simulink model "internalights"  (R2020b)
settings: Solver=FixedStepAuto  StartTime=0.0  StopTime=10  FixedStep=0.1  RelTol=1e-3
undefined symbols (not defined in the file): sigbuilder_block
libraries: simulink x4
settings Model: NumberOfSteps=10  Creator=training  LastModifiedBy=training

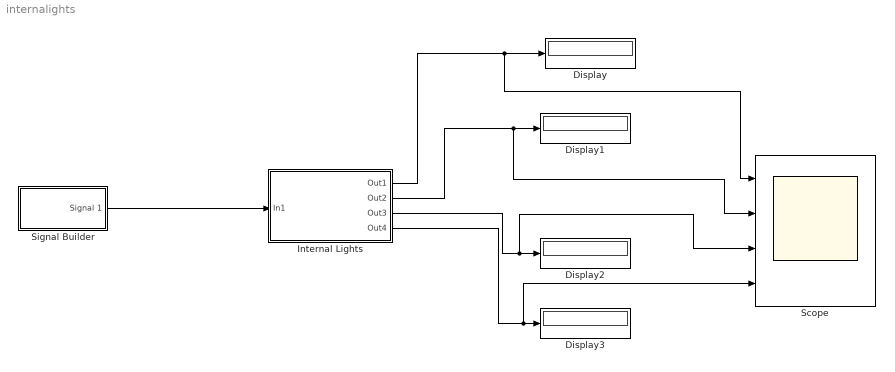
== system internalights ==
  Display{,1..3} (4 alike) : Display
  Internal Lights : Subsystem
  Scope : Scope  NumInputPorts=4
  Signal Builder : Subsystem  Tag=STV Subsys  LoadFcn=sigbuilder_block('load');  StartFcn=sigbuilder_block('start');  StopFcn=sigbuilder_block('stop');  ClipboardFcn=sigbuilder_block('clipboard');  mask(Sigbuilder block){tuvar=[0:10]}
      mask help: Simulink:masks:SigbuilderBlock_MD
      mask init:
      | if ~strcmp(get_param(bdroot(gcbh),'SimulationStatus'),'stopped') tuvar = sigbuilder_block('maskInit'); end
      settings: CopyFcn=sigbuilder_block('copy');  DeleteFcn=sigbuilder_block('delete');  ModelCloseFcn=sigbuilder_block('modelClose');  PreSaveFcn=sigbuilder_block('preSave');  PauseFcn=sigbuilder_block('pause');  ContinueFcn=sigbuilder_block('continue');  NameChangeFcn=sigbuilder_block('namechange');  OpenFcn=sigbuilder_block('open',[437.6 153 550.4 359.25 ]);  CloseFcn=sigbuilder_block('close');
      mask Display: plot(0, 0, 100, 100,[2, 2, 32, 32, 2], [68, 8, 8, 68, 68],[32, 2], [38, 38], [32, 19, 2],[53, 60, 44], [32, 17, 17, 2],[16, 16, 31, 31]);txt = getActiveGroup(gcbh);text(2, 100, txt,'verticalAlignment', 'top');
  wires:
  Signal Builder/1(Signal 1) -> Internal Lights/1(In1)
  Internal Lights/1(Out1) -> Scope/1, Display/1
  Internal Lights/2(Out2) -> Scope/2, Display1/1
  Internal Lights/3(Out3) -> Scope/3, Display2/1
  Internal Lights/4(Out4) -> Scope/4, Display3/1

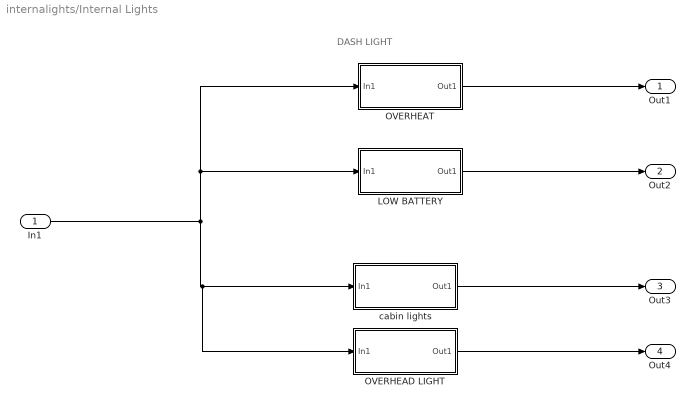
== system internalights/Internal Lights ==
  note: DASH LIGHT
  In1 : Inport
  LOW BATTERY : Subsystem
  OVERHEAD LIGHT : Subsystem
  OVERHEAT : Subsystem
  cabin lights : Subsystem
  Out1 : Outport
  Out2 : Outport  Port=2
  Out3 : Outport  Port=3
  Out4 : Outport  Port=4
  wires:
  In1/1 -> OVERHEAD LIGHT/1(In1), cabin lights/1(In1), LOW BATTERY/1(In1), OVERHEAT/1(In1)
  OVERHEAT/1(Out1) -> Out1/1
  LOW BATTERY/1(Out1) -> Out2/1
  OVERHEAD LIGHT/1(Out1) -> Out4/1
  cabin lights/1(Out1) -> Out3/1

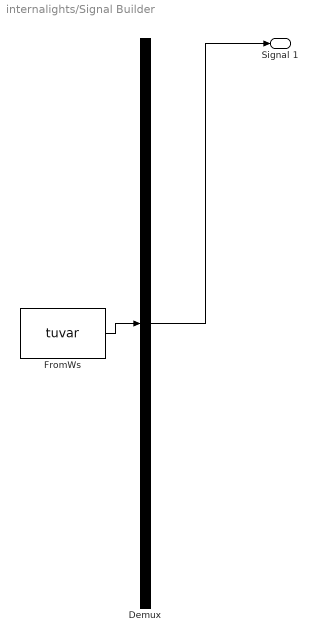
== system internalights/Signal Builder ==
  Demux : Demux  Tag=STV Demux  Outputs=1
      settings: DisplayOption=none
  FromWs : FromWorkspace  Tag=STV FromWs  VariableName=tuvar
      SigBuilderData=|
      | common.afterFinalStr = 'Extrapolate'
      | common.sampleTime = 0
      | dataSet.timeRange = [0 10]
      | dataSet.name = 'Group 1'
      | sbobj.Groups.Name = 'Group 1'
      | sbobj.Groups.Signals.Name = 'Signal 1'
      | sbobj.Groups.Signals.XData = [0 4 4 6 6 10]
      | sbobj.Groups.Signals.YData = [0 0 1 1 0 0]
  Signal 1 : Outport  Tag=STV Outport
  wires:
  Demux/1 -> Signal 1/1
  FromWs/1 -> Demux/1

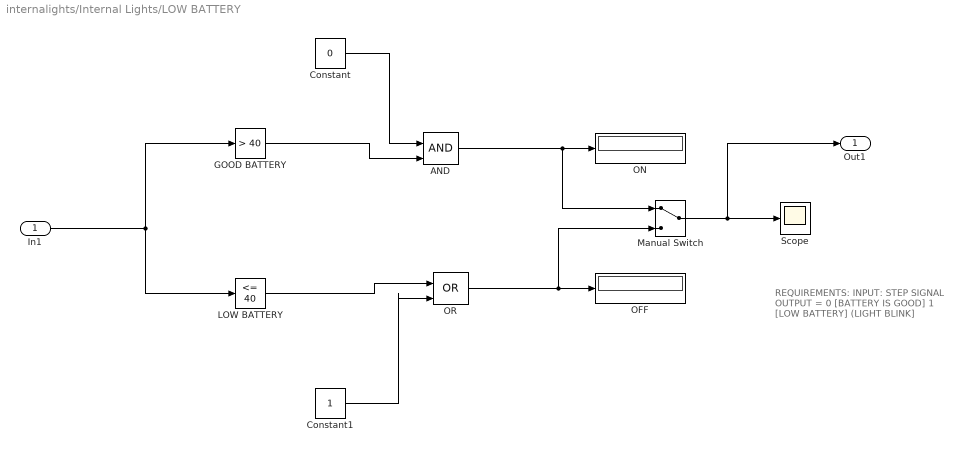
== system internalights/Internal Lights/LOW BATTERY ==
  note: REQUIREMENTS:
      | INPUT: STEP SIGNAL
      | OUTPUT = 0 [BATTERY IS GOOD]
      | 1 [LOW BATTERY] (LIGHT BLINK]
  In1 : Inport
  AND : Logic  IconShape=distinctive  AllPortsSameDT=off  OutDataTypeStr=boolean
  Constant : Constant  Value=0
  Constant1 : Constant
  GOOD BATTERY : simulink/Logic and Bit Operations/Compare To Constant  relop=>  const=40  OutDataTypeStr=boolean
  LOW BATTERY : simulink/Logic and Bit Operations/Compare To Constant  relop=<=  const=40  OutDataTypeStr=boolean
  Manual Switch : ManualSwitch
  OFF : Display
  ON : Display
  OR : Logic  Operator=OR  IconShape=distinctive  AllPortsSameDT=off  OutDataTypeStr=boolean
  Scope : Scope
  Out1 : Outport
  wires:
  OR/1 -> Manual Switch/2, OFF/1
  AND/1 -> Manual Switch/1, ON/1
  Manual Switch/1 -> Out1/1, Scope/1
  Constant1/1 -> OR/2
  GOOD BATTERY/1 -> AND/2
  Constant/1 -> AND/1
  LOW BATTERY/1 -> OR/1
  In1/1 -> LOW BATTERY/1, GOOD BATTERY/1

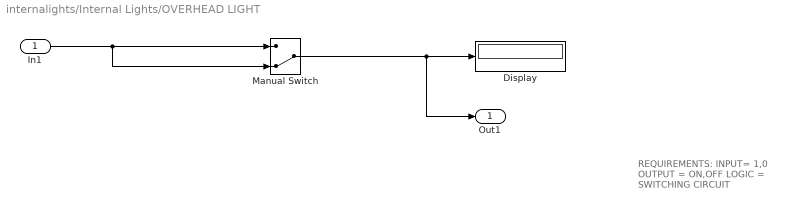
== system internalights/Internal Lights/OVERHEAD LIGHT ==
  note: REQUIREMENTS:
      | INPUT= 1,0
      | OUTPUT = ON,OFF
      | LOGIC = SWITCHING CIRCUIT
  In1 : Inport
  Display : Display
  Manual Switch : ManualSwitch  CurrentSetting=0
  Out1 : Outport
  wires:
  In1/1 -> Manual Switch/2, Manual Switch/1
  Manual Switch/1 -> Out1/1, Display/1

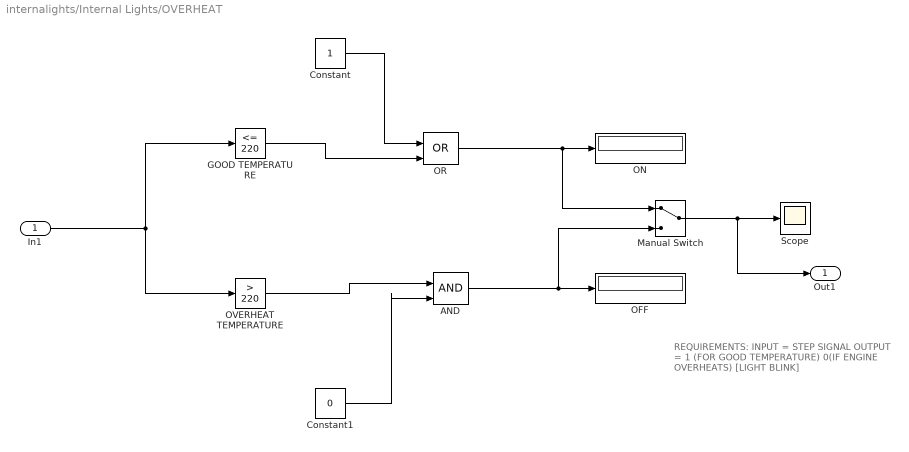
== system internalights/Internal Lights/OVERHEAT ==
  note: REQUIREMENTS:
      | INPUT = STEP SIGNAL
      | OUTPUT = 1 (FOR GOOD TEMPERATURE)
      | 0(IF ENGINE OVERHEATS) [LIGHT BLINK]
  In1 : Inport
  AND : Logic  IconShape=distinctive  AllPortsSameDT=off  OutDataTypeStr=boolean
  Constant : Constant
  Constant1 : Constant  Value=0
  GOOD TEMPERATURE : simulink/Logic and Bit Operations/Compare To Constant  relop=<=  const=220  OutDataTypeStr=boolean
  Manual Switch : ManualSwitch
  OFF : Display
  ON : Display
  OR : Logic  Operator=OR  IconShape=distinctive  AllPortsSameDT=off  OutDataTypeStr=boolean
  OVERHEAT TEMPERATURE : simulink/Logic and Bit Operations/Compare To Constant  relop=>  const=220  OutDataTypeStr=boolean
  Scope : Scope
  Out1 : Outport
  wires:
  In1/1 -> OVERHEAT TEMPERATURE/1, GOOD TEMPERATURE/1
  Constant/1 -> OR/1
  GOOD TEMPERATURE/1 -> OR/2
  OVERHEAT TEMPERATURE/1 -> AND/1
  Constant1/1 -> AND/2
  OR/1 -> Manual Switch/1, ON/1
  AND/1 -> Manual Switch/2, OFF/1
  Manual Switch/1 -> Out1/1, Scope/1

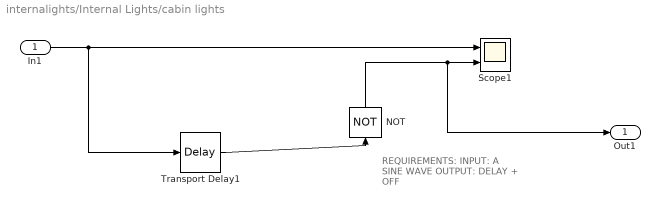
== system internalights/Internal Lights/cabin lights ==
  note: REQUIREMENTS:
      | INPUT: A SINE WAVE
      | OUTPUT: DELAY + OFF
  In1 : Inport
  NOT : Logic  Operator=NOT  AllPortsSameDT=off  OutDataTypeStr=boolean
  Scope1 : Scope  NumInputPorts=2
  Transport Delay1 : TransportDelay  DelayTime=3
  Out1 : Outport
  wires:
  Transport Delay1/1 -> NOT/1
  NOT/1 -> Out1/1, Scope1/2
  In1/1 -> Scope1/1, Transport Delay1/1
